simulink library "library"  (R2017a)
settings: Solver=VariableStepAuto  StartTime=0.0  StopTime=10.0  RelTol=1e-3
undefined symbols (not defined in the file or in its folder): gcbh, sps_rtmsupport
libraries: powerlib x31, spsVIMeasurementModel x27, sps_avr x3, powerlib_meascontrol x2, library x1
(part 2 of 2)

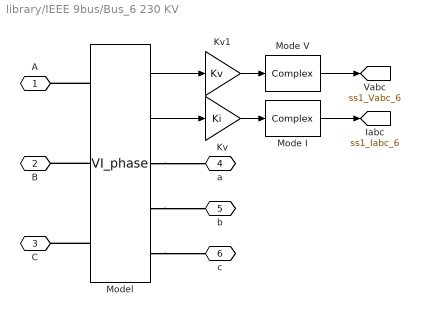
== system library/IEEE 9bus/Bus_6 230 KV ==
  Kv : Gain  Gain=Ki  SaturateOnIntegerOverflow=on  OutDataTypeStr=Inherit: Same as input  ParamDataTypeStr=Inherit: Same as input
  Kv1 : Gain  Gain=Kv  SaturateOnIntegerOverflow=on  OutDataTypeStr=Inherit: Same as input  ParamDataTypeStr=Inherit: Same as input
  Mode I : spsVIMeasurementModel/Complex
  Mode V : spsVIMeasurementModel/Complex
  Model : spsVIMeasurementModel/VI_phase  SystemSampleTime=-1
  A : PMIOPort  Port=1  Side=Left
  B : PMIOPort  Port=2  Side=Left
  C : PMIOPort  Port=3  Side=Left
  a : PMIOPort  Port=4  Side=Right
  b : PMIOPort  Port=5  Side=Right
  c : PMIOPort  Port=6  Side=Right
  tag scope: ss1_Iabc_6=global, ss1_Vabc_6=global
  wires:
  Model/2 -> Kv/1
  Model/1 -> Kv1/1
  Kv/1 -> Mode I/1
  Kv1/1 -> Mode V/1
  Mode I/1 -> [ss1_Iabc_6]
  Mode V/1 -> [ss1_Vabc_6]
  connections:
  Model/RConn3 -- c/RConn1
  Model/RConn1 -- a/RConn1
  Model/RConn2 -- b/RConn1
  Model/LConn3 -- C/RConn1
  Model/LConn1 -- A/RConn1
  Model/LConn2 -- B/RConn1

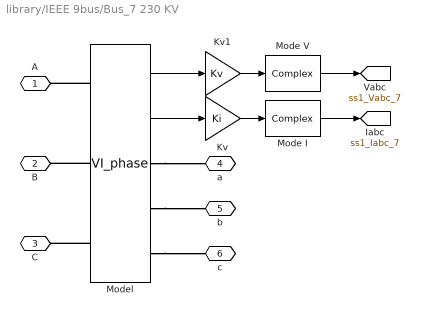
== system library/IEEE 9bus/Bus_7 230 KV  ==
  Kv : Gain  Gain=Ki  SaturateOnIntegerOverflow=on  OutDataTypeStr=Inherit: Same as input  ParamDataTypeStr=Inherit: Same as input
  Kv1 : Gain  Gain=Kv  SaturateOnIntegerOverflow=on  OutDataTypeStr=Inherit: Same as input  ParamDataTypeStr=Inherit: Same as input
  Mode I : spsVIMeasurementModel/Complex
  Mode V : spsVIMeasurementModel/Complex
  Model : spsVIMeasurementModel/VI_phase  SystemSampleTime=-1
  A : PMIOPort  Port=1  Side=Left
  B : PMIOPort  Port=2  Side=Left
  C : PMIOPort  Port=3  Side=Left
  a : PMIOPort  Port=4  Side=Right
  b : PMIOPort  Port=5  Side=Right
  c : PMIOPort  Port=6  Side=Right
  tag scope: ss1_Iabc_7=global, ss1_Vabc_7=global
  wires:
  Model/2 -> Kv/1
  Model/1 -> Kv1/1
  Kv/1 -> Mode I/1
  Kv1/1 -> Mode V/1
  Mode I/1 -> [ss1_Iabc_7]
  Mode V/1 -> [ss1_Vabc_7]
  connections:
  Model/RConn3 -- c/RConn1
  Model/RConn1 -- a/RConn1
  Model/RConn2 -- b/RConn1
  Model/LConn3 -- C/RConn1
  Model/LConn1 -- A/RConn1
  Model/LConn2 -- B/RConn1

== system library/IEEE 9bus/Bus_8 230 KV ==
  Kv : Gain  Gain=Ki  SaturateOnIntegerOverflow=on  OutDataTypeStr=Inherit: Same as input  ParamDataTypeStr=Inherit: Same as input
  Kv1 : Gain  Gain=Kv  SaturateOnIntegerOverflow=on  OutDataTypeStr=Inherit: Same as input  ParamDataTypeStr=Inherit: Same as input
  Mode I : spsVIMeasurementModel/Complex
  Mode V : spsVIMeasurementModel/Complex
  Model : spsVIMeasurementModel/VI_phase  SystemSampleTime=-1
  A : PMIOPort  Port=1  Side=Left
  B : PMIOPort  Port=2  Side=Left
  C : PMIOPort  Port=3  Side=Left
  a : PMIOPort  Port=4  Side=Right
  b : PMIOPort  Port=5  Side=Right
  c : PMIOPort  Port=6  Side=Right
  tag scope: ss1_Iabc_8=global, ss1_Vabc_8=global
  wires:
  Model/2 -> Kv/1
  Model/1 -> Kv1/1
  Kv/1 -> Mode I/1
  Kv1/1 -> Mode V/1
  Mode I/1 -> [ss1_Iabc_8]
  Mode V/1 -> [ss1_Vabc_8]
  connections:
  Model/RConn3 -- c/RConn1
  Model/RConn1 -- a/RConn1
  Model/RConn2 -- b/RConn1
  Model/LConn3 -- C/RConn1
  Model/LConn1 -- A/RConn1
  Model/LConn2 -- B/RConn1

== system library/IEEE 9bus/Bus_9 230 KV ==
  Kv : Gain  Gain=Ki  SaturateOnIntegerOverflow=on  OutDataTypeStr=Inherit: Same as input  ParamDataTypeStr=Inherit: Same as input
  Kv1 : Gain  Gain=Kv  SaturateOnIntegerOverflow=on  OutDataTypeStr=Inherit: Same as input  ParamDataTypeStr=Inherit: Same as input
  Mode I : spsVIMeasurementModel/Complex
  Mode V : spsVIMeasurementModel/Complex
  Model : spsVIMeasurementModel/VI_phase  SystemSampleTime=-1
  A : PMIOPort  Port=1  Side=Left
  B : PMIOPort  Port=2  Side=Left
  C : PMIOPort  Port=3  Side=Left
  a : PMIOPort  Port=4  Side=Right
  b : PMIOPort  Port=5  Side=Right
  c : PMIOPort  Port=6  Side=Right
  tag scope: ss1_Iabc_9=global, ss1_Vabc_9=global
  wires:
  Model/2 -> Kv/1
  Model/1 -> Kv1/1
  Kv/1 -> Mode I/1
  Kv1/1 -> Mode V/1
  Mode I/1 -> [ss1_Iabc_9]
  Mode V/1 -> [ss1_Vabc_9]
  connections:
  Model/RConn3 -- c/RConn1
  Model/RConn1 -- a/RConn1
  Model/RConn2 -- b/RConn1
  Model/LConn3 -- C/RConn1
  Model/LConn1 -- A/RConn1
  Model/LConn2 -- B/RConn1

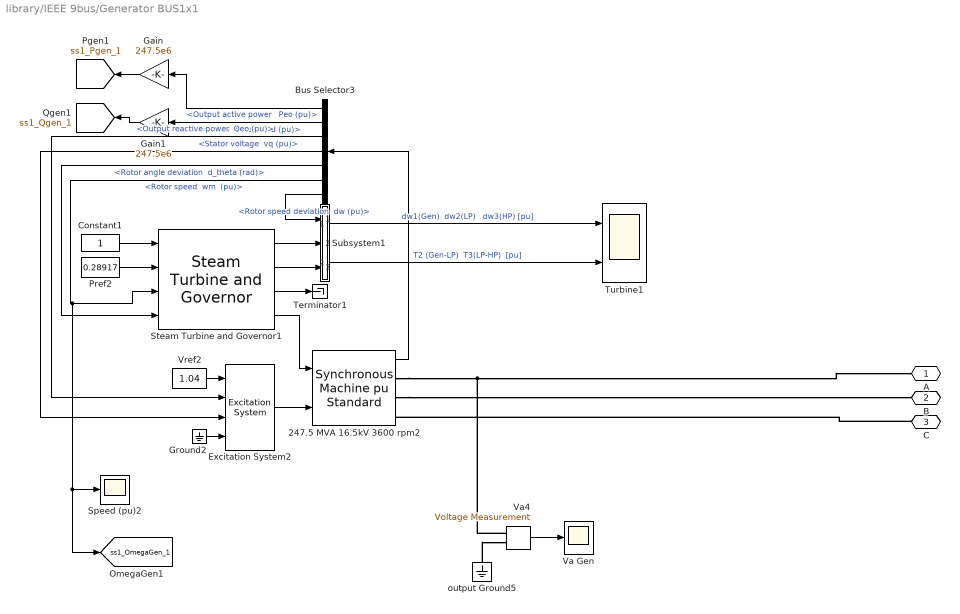
== system library/IEEE 9bus/Generator BUS1x1 ==
  " Speed (pu)2" : Scope
  247.5 MVA 16.5kV 3600 rpm2 : powerlib/Machines/Synchronous Machine pu Standard  PresetModel=No  MechanicalLoad=Mechanical power Pm  ShowDetailedParameters=on  RotorType=Round  Units=per unit standard parameters  MeasurementBus=off  NominalParameters="[ 247.5e6  16.5e3   60 ]"  Reactances1=[ 0.36135, 0.15048, 0.12375, 0.2475, 0.2398275, 0.12375, 0.08316 ]  Reactances2="[ 1.305, 0.296, 0.252, 0.474,  0.243,  0.18 ]"  dAxisTimeConstants=Open-circuit  qAxisTimeConstants=Open-circuit  TimeConstants1="[ 4.4849  0.0681  0.1  ]"  TimeConstants2="[ 8.96, 0.05,  0.31, 0.05 ]"  TimeConstants3="[  4.49  0.0681  0.0513  ]"  TimeConstants4=[ 8.0, 0.03, 0.3371, 0.0295 ]  TimeConstants5=[ 1.01, 0.053, 0.1 ]  TimeConstants6=[ 1.3201, 0.023, 1.0, 0.07 ]  TimeConstants7="[  1.01  0.053  0.051266  ]"  TimeConstants8=[ 1.3201, 0.0231, 0.3371, 0.0295 ]  StatorResistance=0.000125  Mechanical="[ 23.64  0 1 ]"  PolePairs=1  InitialConditions=[0 -86.3058 0.296671 0.296671 0.296671 -20.4087 -140.409 99.5913 1.08165]  SetSaturation=off  Saturation=[0.6404,0.7127,0.8441,0.9214,0.9956,1.082,1.19,1.316,1.457;0.7,0.7698,0.8872,0.9466,0.9969,1.046,1.1,1.151,1.201]  LoadFlowParameters=[2 71600000 0 0 0]  TsPowergui=0  TsBlock=-1  IterativeModel=Trapezoidal non iterative  IterativeDiscreteModel=Trapezoidal non iterative  BusType=swing  Pref=0  Qref=0  Qmin=-Inf  Qmax=Inf  PLF=0  QLF=0
      settings: SourceProductName=Simscape Power Systems
  Bus Selector3 : BusSelector  OutputSignals="Output active power   Peo (pu),Output reactive power  Qeo (pu),dq0 components.Stator voltage  vd (pu),dq0 components.Stator voltage  vq (pu),Mechanical.Rotor angle deviation  d_theta (rad),Mechanical.Rotor speed  wm  (pu),Mechanical.Rotor speed deviation  dw (pu)"
  Constant1 : Constant
  Excitation System2 : sps_avr/Excitation System  tr=20e-3  reg=[ 200, 0.02 ]  exc=[ 1, 0 ]  tgr=[ 12.0, 1.0 ]  damp=[ 0.03, 1.0 ]  sat=[ 0, 0 ]  lim=[ -10.0, 10.0, 0 ]  v0=[1.04 1.0817]
      settings: SourceProductName=Simscape Power Systems  SourceProductBaseCode=PS
  Gain : Gain  Gain=247.5e6
  Gain1 : Gain  Gain=247.5e6
  Ground2 : Ground
  Pref2 : Constant  Value=0.28917
  Steam Turbine and Governor1 : powerlib/Machines/Steam Turbine and Governor  gentype=Tandem-compound (single mass)  reg1="[ 1  0.05    0 ]"  reg2="[ 0.001  0.1 ]"  reg3="[ -10.0 0.1   0.1 1.0 ]"  N=3600  turb1="[ 0.12  0.13  10.0   0.32   ]"  turb2="[ 0.48   0.25   0  0.27 ]"  HA="[  1.5498   0.24894  0  0 ]"  KA="[  83.47  42.702  0  0 ]"  DA="[  0.3104  0.05  0  0 ]*8"  ini1=0.28918  ini2=[1.88924e-008,-120.067]
      settings: SourceProductName=Simscape Power Systems  SourceProductBaseCode=PS
  Subsystem1 : Subsystem
  Terminator1 : Terminator
  Turbine1 : Scope  NumInputPorts=2
  Va Gen : Scope
  Va4 : powerlib/Measurements/Voltage Measurement  Tag=PoWeRsYsTeMmEaSuReMeNt  PhasorSimulation=off  OutputType=Magnitude  PSBequivalent=0
  Vref2 : Constant  Value=1.04
  output Ground5 : powerlib/Elements/Ground  LConnTagsString=a
  A : PMIOPort  Port=1  Side=Right
  B : PMIOPort  Port=2  Side=Right
  C : PMIOPort  Port=3  Side=Right
  tag scope: ss1_OmegaGen_1=global, ss1_Pgen_1=global, ss1_Qgen_1=global
  wires:
  Constant1/1 -> Steam Turbine and Governor1/1
  Bus Selector3/5 -> Steam Turbine and Governor1/4  "<Rotor angle deviation  d_theta (rad)>"
  Subsystem1/2(T_23) -> Turbine1/2  "T2 (Gen-LP)  T3(LP-HP)  [pu]"
  Steam Turbine and Governor1/3 -> Terminator1/1
  Bus Selector3/7 -> Subsystem1/1(In1)  "<Rotor speed deviation  dw (pu)>"
  Vref2/1 -> Excitation System2/1
  Pref2/1 -> Steam Turbine and Governor1/2
  Steam Turbine and Governor1/1 -> Subsystem1/2(In2)
  Subsystem1/1(dw_123) -> Turbine1/1  "dw1(Gen)  dw2(LP)   dw3(HP) [pu]"
  Steam Turbine and Governor1/4 -> 247.5 MVA 16.5kV 3600 rpm2/1
  Steam Turbine and Governor1/2 -> Subsystem1/3(In3)
  Bus Selector3/6 -> [ss1_OmegaGen_1], " Speed (pu)2"/1, Steam Turbine and Governor1/3  "<Rotor speed  wm  (pu)>"
  247.5 MVA 16.5kV 3600 rpm2/1 -> Bus Selector3/1
  Ground2/1 -> Excitation System2/4
  Bus Selector3/4 -> Excitation System2/3  "<Stator voltage  vq (pu)>"
  Bus Selector3/3 -> Excitation System2/2  "<Stator voltage  vd (pu)>"
  Excitation System2/1 -> 247.5 MVA 16.5kV 3600 rpm2/2
  Va4/1 -> Va Gen/1
  Bus Selector3/1 -> Gain/1  "<Output active power   Peo (pu)>"
  Bus Selector3/2 -> Gain1/1  "<Output reactive power  Qeo (pu)>"
  Gain/1 -> [ss1_Pgen_1]
  Gain1/1 -> [ss1_Qgen_1]
  connections:
  output Ground5/LConn1 -- Va4/LConn2
  C/RConn1 -- 247.5 MVA 16.5kV 3600 rpm2/RConn3
  247.5 MVA 16.5kV 3600 rpm2/RConn2 -- B/RConn1
  Va4/LConn1 -- 247.5 MVA 16.5kV 3600 rpm2/RConn1 -- A/RConn1

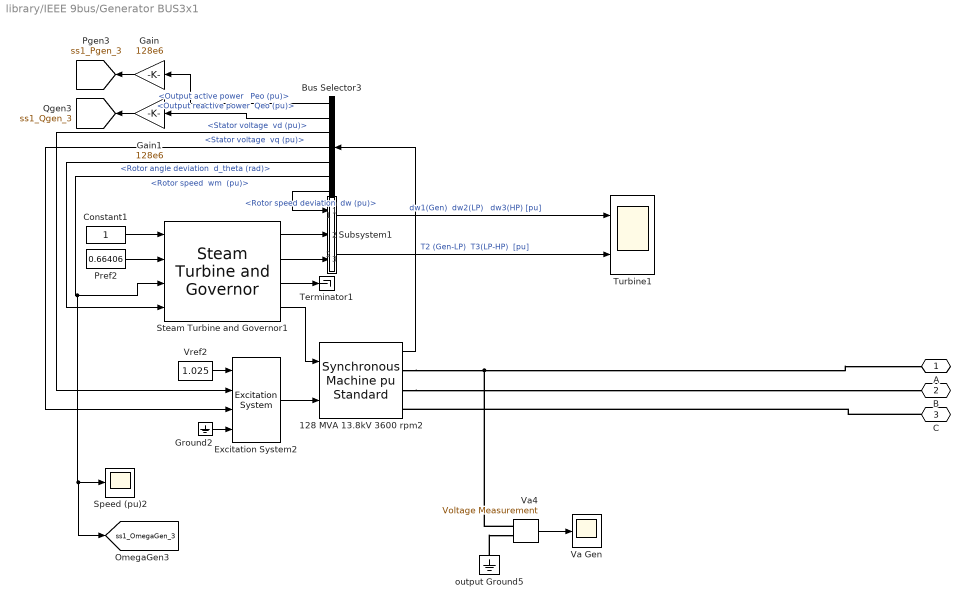
== system library/IEEE 9bus/Generator BUS3x1 ==
  " Speed (pu)2" : Scope
  128 MVA 13.8kV 3600 rpm2 : powerlib/Machines/Synchronous Machine pu Standard  PresetModel=No  MechanicalLoad=Mechanical power Pm  ShowDetailedParameters=on  RotorType=Round  Units=per unit standard parameters  MeasurementBus=off  NominalParameters="[ 128e6  13.8e3   60 ]"  Reactances1=[ 1.68, 0.232064, 0.1536, 1.609984, 0.32, 0.2176, 0.094976 ]  Reactances2="[ 1.305, 0.296, 0.252, 0.474,  0.243,  0.18 ]"  dAxisTimeConstants=Open-circuit  qAxisTimeConstants=Open-circuit  TimeConstants1="[ 4.4849  0.0681  0.1  ]"  TimeConstants2="[ 5.89, 0.05,  0.6, 0.05 ]"  TimeConstants3="[  4.49  0.0681  0.0513  ]"  TimeConstants4=[ 8.0, 0.03, 0.3371, 0.0295 ]  TimeConstants5=[ 1.01, 0.053, 0.1 ]  TimeConstants6=[ 1.3201, 0.023, 1.0, 0.07 ]  TimeConstants7="[  1.01  0.053  0.051266  ]"  TimeConstants8=[ 1.3201, 0.0231, 0.3371, 0.0295 ]  StatorResistance=0.000125  Mechanical="[ 3.01  0 1 ]"  PolePairs=1  InitialConditions=[0 -35.8791 0.653244 0.653244 0.653244 11.9635 -108.037 131.963 1.40212]  SetSaturation=off  Saturation=[0.6404,0.7127,0.8441,0.9214,0.9956,1.082,1.19,1.316,1.457;0.7,0.7698,0.8872,0.9466,0.9969,1.046,1.1,1.151,1.201]  LoadFlowParameters=[1 85000000 0 0 0]  TsPowergui=0  TsBlock=-1  IterativeModel=Trapezoidal non iterative  IterativeDiscreteModel=Trapezoidal non iterative  BusType=PV  Pref=85e6  Qref=0  Qmin=-Inf  Qmax=Inf  PLF=0  QLF=0
      settings: SourceProductName=Simscape Power Systems
  Bus Selector3 : BusSelector  OutputSignals="Output active power   Peo (pu),Output reactive power  Qeo (pu),dq0 components.Stator voltage  vd (pu),dq0 components.Stator voltage  vq (pu),Mechanical.Rotor angle deviation  d_theta (rad),Mechanical.Rotor speed  wm  (pu),Mechanical.Rotor speed deviation  dw (pu)"
  Constant1 : Constant
  Excitation System2 : sps_avr/Excitation System  tr=20e-3  reg=[ 200, 0.02 ]  exc=[ 1, 0 ]  tgr=[ 12.0, 1.0 ]  damp=[ 0.03, 1.0 ]  sat=[ 0, 0 ]  lim=[ -10.0, 10.0, 0 ]  v0=[1.025 1.4021]
      settings: SourceProductName=Simscape Power Systems  SourceProductBaseCode=PS
  Gain : Gain  Gain=128e6
  Gain1 : Gain  Gain=128e6
  Ground2 : Ground
  Pref2 : Constant  Value=0.66406
  Steam Turbine and Governor1 : powerlib/Machines/Steam Turbine and Governor  gentype=Tandem-compound (single mass)  reg1="[ 1  0.05    0 ]"  reg2="[ 0.001  0.1 ]"  reg3="[ -10.0 0.1   0.1 1.0 ]"  N=3600  turb1="[ 0.12  0.13  10.0   0.32   ]"  turb2="[ 0.48   0.25   0  0.27 ]"  HA="[  1.5498   0.24894  0  0 ]"  KA="[  83.47  42.702  0  0 ]"  DA="[  0.3104  0.05  0  0 ]*8"  ini1=0.66412  ini2=[1.88924e-008,-120.067]
      settings: SourceProductName=Simscape Power Systems  SourceProductBaseCode=PS
  Subsystem1 : Subsystem
  Terminator1 : Terminator
  Turbine1 : Scope  NumInputPorts=2
  Va Gen : Scope
  Va4 : powerlib/Measurements/Voltage Measurement  Tag=PoWeRsYsTeMmEaSuReMeNt  PhasorSimulation=off  OutputType=Magnitude  PSBequivalent=0
  Vref2 : Constant  Value=1.025
  output Ground5 : powerlib/Elements/Ground  LConnTagsString=a
  A : PMIOPort  Port=1  Side=Right
  B : PMIOPort  Port=2  Side=Right
  C : PMIOPort  Port=3  Side=Right
  tag scope: ss1_OmegaGen_3=global, ss1_Pgen_3=global, ss1_Qgen_3=global
  wires:
  Constant1/1 -> Steam Turbine and Governor1/1
  Bus Selector3/5 -> Steam Turbine and Governor1/4  "<Rotor angle deviation  d_theta (rad)>"
  Subsystem1/2(T_23) -> Turbine1/2  "T2 (Gen-LP)  T3(LP-HP)  [pu]"
  Steam Turbine and Governor1/3 -> Terminator1/1
  Bus Selector3/7 -> Subsystem1/1(In1)  "<Rotor speed deviation  dw (pu)>"
  Vref2/1 -> Excitation System2/1
  Pref2/1 -> Steam Turbine and Governor1/2
  Steam Turbine and Governor1/1 -> Subsystem1/2(In2)
  Subsystem1/1(dw_123) -> Turbine1/1  "dw1(Gen)  dw2(LP)   dw3(HP) [pu]"
  Steam Turbine and Governor1/4 -> 128 MVA 13.8kV 3600 rpm2/1
  Steam Turbine and Governor1/2 -> Subsystem1/3(In3)
  Bus Selector3/6 -> [ss1_OmegaGen_3], " Speed (pu)2"/1, Steam Turbine and Governor1/3  "<Rotor speed  wm  (pu)>"
  128 MVA 13.8kV 3600 rpm2/1 -> Bus Selector3/1
  Ground2/1 -> Excitation System2/4
  Bus Selector3/4 -> Excitation System2/3  "<Stator voltage  vq (pu)>"
  Bus Selector3/3 -> Excitation System2/2  "<Stator voltage  vd (pu)>"
  Excitation System2/1 -> 128 MVA 13.8kV 3600 rpm2/2
  Va4/1 -> Va Gen/1
  Gain/1 -> [ss1_Pgen_3]
  Bus Selector3/1 -> Gain/1  "<Output active power   Peo (pu)>"
  Gain1/1 -> [ss1_Qgen_3]
  Bus Selector3/2 -> Gain1/1  "<Output reactive power  Qeo (pu)>"
  connections:
  output Ground5/LConn1 -- Va4/LConn2
  C/RConn1 -- 128 MVA 13.8kV 3600 rpm2/RConn3
  128 MVA 13.8kV 3600 rpm2/RConn2 -- B/RConn1
  Va4/LConn1 -- 128 MVA 13.8kV 3600 rpm2/RConn1 -- A/RConn1

== system library/IEEE 9bus/Generator BUS1x1/Subsystem1 ==
  In1 : Inport
  In2 : Inport  Port=2
  In3 : Inport  Port=3
  Gain : Gain  Gain=-1  SaturateOnIntegerOverflow=on  OutDataTypeStr=Inherit: Same as input  ParamDataTypeStr=Inherit: Same as input
  Mux : Mux  Inputs=2
  Selector : Selector  InputPortWidth=4  IndexOptions=Index vector (dialog)  Indices=[4 3]  OutputSizes=1
  Selector1 : Selector  InputPortWidth=4  IndexOptions=Index vector (dialog)  Indices=[4 3]  OutputSizes=1
  dw_123 : Outport
  T_23 : Outport  Port=2
  wires:
  Selector/1 -> Mux/2
  Mux/1 -> dw_123/1
  In1/1 -> Mux/1
  In2/1 -> Selector/1
  In3/1 -> Selector1/1
  Selector1/1 -> Gain/1
  Gain/1 -> T_23/1

== system library/IEEE 9bus/Generator BUS3x1/Subsystem1 ==
  In1 : Inport
  In2 : Inport  Port=2
  In3 : Inport  Port=3
  Gain : Gain  Gain=-1  SaturateOnIntegerOverflow=on  OutDataTypeStr=Inherit: Same as input  ParamDataTypeStr=Inherit: Same as input
  Mux : Mux  Inputs=2
  Selector : Selector  InputPortWidth=4  IndexOptions=Index vector (dialog)  Indices=[4 3]  OutputSizes=1
  Selector1 : Selector  InputPortWidth=4  IndexOptions=Index vector (dialog)  Indices=[4 3]  OutputSizes=1
  dw_123 : Outport
  T_23 : Outport  Port=2
  wires:
  Selector/1 -> Mux/2
  Mux/1 -> dw_123/1
  In1/1 -> Mux/1
  In2/1 -> Selector/1
  In3/1 -> Selector1/1
  Selector1/1 -> Gain/1
  Gain/1 -> T_23/1
